simulink model "CTRL_LO_ST1_YAWTRQLAT_test"  (R2023b)
settings: Solver=VariableStepAuto  StartTime=0.0  StopTime=10.0  RelTol=1e-3
libraries: CTRL_LO_ST1_YAWTRQLAT x1
settings Model: Creator=blatak  LastModifiedBy=blatak

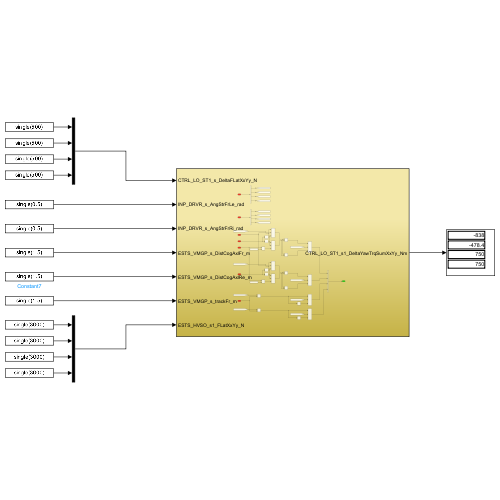
[thumbnail: Simulink's stored preview of the top-level diagram]
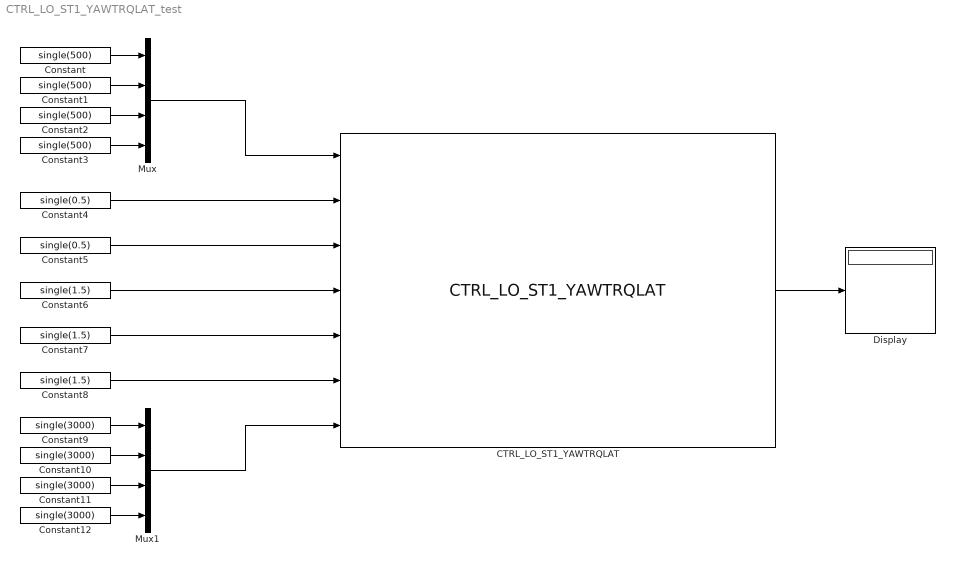
== system CTRL_LO_ST1_YAWTRQLAT_test ==
  CTRL_LO_ST1_YAWTRQLAT : CTRL_LO_ST1_YAWTRQLAT/CTRL_LO_ST1_YAWTRQLAT  SystemSampleTime=-1  VariantActivationTime=update diagram  AllowFlexibleInterface=on  Latency=0  AutoFrameSizeCalculation=off
  Constant{,1..3} (4 alike) : Constant  Value=single(500)
  Constant{9..12} (4 alike) : Constant  Value=single(3000)
  Constant4 : Constant  Value=single(0.5)
  Constant5 : Constant  Value=single(0.5)
  Constant6 : Constant  Value=single(1.5)
  Constant7 : Constant  Value=single(1.5)
  Constant8 : Constant  Value=single(1.5)
  Display : Display
  Mux : Mux
  Mux1 : Mux
  wires:
  Constant/1 -> Mux/1
  Constant1/1 -> Mux/2
  Constant3/1 -> Mux/4
  Constant2/1 -> Mux/3
  Mux/1 -> CTRL_LO_ST1_YAWTRQLAT/1
  Constant4/1 -> CTRL_LO_ST1_YAWTRQLAT/2
  Constant5/1 -> CTRL_LO_ST1_YAWTRQLAT/3
  Constant6/1 -> CTRL_LO_ST1_YAWTRQLAT/4
  Constant7/1 -> CTRL_LO_ST1_YAWTRQLAT/5
  Constant8/1 -> CTRL_LO_ST1_YAWTRQLAT/6
  Constant10/1 -> Mux1/2
  Constant9/1 -> Mux1/1
  Constant11/1 -> Mux1/3
  Constant12/1 -> Mux1/4
  Mux1/1 -> CTRL_LO_ST1_YAWTRQLAT/7
  CTRL_LO_ST1_YAWTRQLAT/1 -> Display/1
